simulink model "Fig38"  (Simulink 8.9)
settings: Solver=ode3  StartTime=0.0  StopTime=10.001  FixedStep=2e-6  RelTol=1e-5  EnableMultiTasking=on
libraries: commfilt2 x1, commchan3 x1, commsink2 x1, commanapbnd3 x1, commrandsrc2 x1
settings Model: Creator=Dennis Silage  LastModifiedBy=Ctu
settings OptimizationCC: ExpressionDepthLimit=2147483647  InitFltsAndDblsToZero=on
settings GRTTargetCC: GeneratePreprocessorConditionals=Use local settings

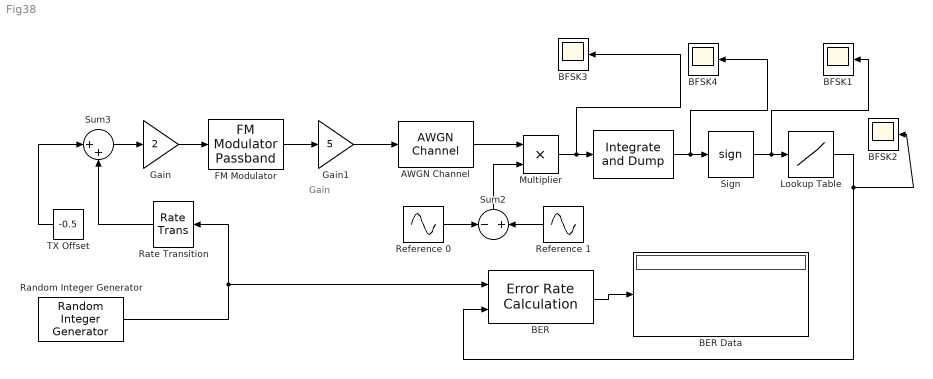
== system Fig38 ==
  note: Gain
  " " : commfilt2/Integrate and Dump  obssamples=500  offsetsamples=0  nodump=off  roundingMode=Floor  overflowMode=off  outputDataTypeStr=Inherit: Same as accumulator  outputLastDataTypeStr=Inherit: Same as accumulator
      settings: SourceProductName=Communications System Toolbox
  AWGN Channel : commchan3/AWGN Channel  InputProcessing=Inherited (this choice will be removed - see release notes)  seed=randseed  noiseMode="Signal to noise ratio  (Eb/No)"  EbNodB=0  EsNodB=10  SNRdB=12  bitsPerSym=1  Ps=25  Tsym=1e-3  variance=0
  BER : commsink2/Error Rate Calculation  N=2  st_delay=0  cp_mode=Entire frame  subframe=[]  PMode=Port  WsName=ErrorVec  RsMode2=off  stop=off  numErr=100  maxBits=1e6
  BER Data : Display
  BFSK{1..4} (4 alike) : Scope
  FM Modulator : commanapbnd3/FM Modulator Passband  Fc=20000  Ph=0  Kc=2000
      settings: SourceProductName=Communications System Toolbox  SourceProductBaseCode=CM
  Gain : Gain  Gain=2
  Gain1 : Gain  Gain=5
  Lookup Table : Lookup  InputValues=[-1,0,1]  Table=[0,0,1]  LookUpMeth=Use Input Nearest
  Multiplier : Product  RndMeth=Zero
  Random Integer Generator : commrandsrc2/Random Integer Generator  mul=2  seed=randseed  Ts=1e-3  frameBased=off  sampPerFrame=50  orient=on  outDataType=double
  Rate Transition : RateTransition  OutPortSampleTime=2e-6
  Reference 0 : Sin  Amplitude=5  Frequency=36000*pi  Phase=pi/2  Samples=200  SampleTime=2e-6
  Reference 1 : Sin  Amplitude=5  Frequency=44000*pi  Phase=pi/2  Samples=200  SampleTime=2e-6
  Sign : Signum
  Sum2 : Sum  Inputs=-+
  Sum3 : Sum  Inputs=|++
  TX Offset : Constant  Value=-0.5
  wires:
  Sign/1 -> BFSK1/1, Lookup Table/1
  BER/1 -> BER Data/1
  Multiplier/1 -> BFSK3/1, " "/1
  Reference 1/1 -> Sum2/2
  Reference 0/1 -> Sum2/1
  " "/1 -> BFSK4/1, Sign/1
  Sum2/1 -> Multiplier/2
  AWGN Channel/1 -> Multiplier/1
  Sum3/1 -> Gain/1
  TX Offset/1 -> Sum3/1
  Rate Transition/1 -> Sum3/2
  Gain/1 -> FM Modulator/1
  FM Modulator/1 -> Gain1/1
  Gain1/1 -> AWGN Channel/1
  Lookup Table/1 -> BFSK2/1, BER/2
  Random Integer Generator/1 -> BER/1, Rate Transition/1
